simulink model "Battery"  (R2018b)
settings: Solver=VariableStepAuto  StartTime=0.0  StopTime=10.0  RelTol=1e-3
settings Model: Creator=jackb  LastModifiedBy=jackb
settings DebuggingCC: LibraryContextMissingDiagnostic=none
settings SFSimCC: SimUseLocalCustomCode=off
settings RTWCC: RTWUseLocalCustomCode=off

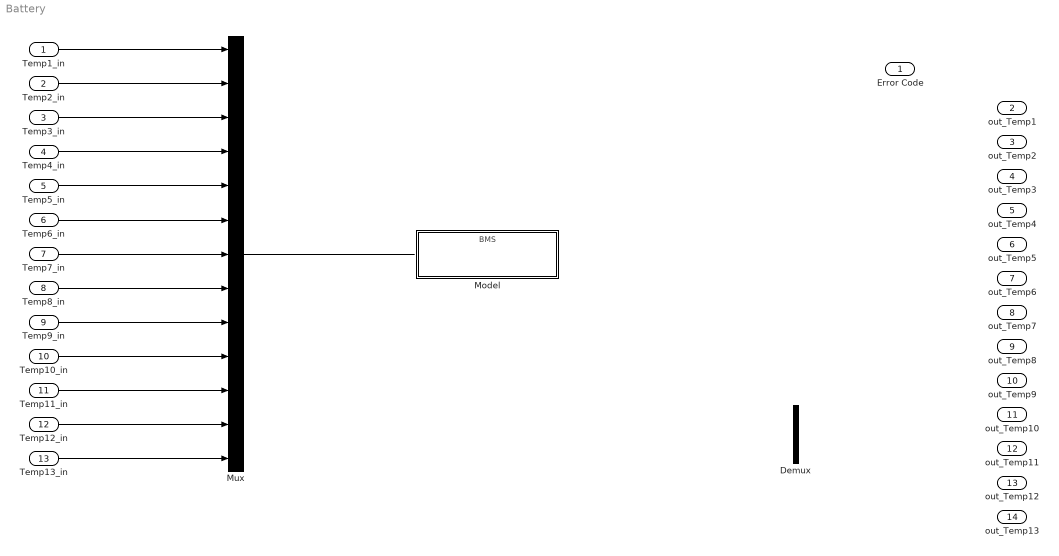
== system Battery ==
  Temp1_in : Inport
  Temp2_in : Inport  Port=2
  "Temp3_in " : Inport  Port=3
  Temp4_in : Inport  Port=4
  Temp5_in : Inport  Port=5
  Temp6_in : Inport  Port=6
  Temp7_in : Inport  Port=7
  Temp8_in : Inport  Port=8
  Temp9_in : Inport  Port=9
  Temp10_in : Inport  Port=10
  Temp11_in : Inport  Port=11
  Temp12_in : Inport  Port=12
  Temp13_in : Inport  Port=13
  Demux : Demux  Outputs=13
  Model : ModelReference  ModelNameDialog=BMS  SimulationMode=Normal
  Mux : Mux  Inputs=13
  Error Code : Outport
  out_Temp1 : Outport  Port=2
  out_Temp2 : Outport  Port=3
  out_Temp3 : Outport  Port=4
  out_Temp4 : Outport  Port=5
  out_Temp5 : Outport  Port=6
  out_Temp6 : Outport  Port=7
  out_Temp7 : Outport  Port=8
  out_Temp8 : Outport  Port=9
  out_Temp9 : Outport  Port=10
  out_Temp10 : Outport  Port=11
  out_Temp11 : Outport  Port=12
  out_Temp12 : Outport  Port=13
  out_Temp13 : Outport  Port=14
  wires:
  Temp1_in/1 -> Mux/1
  Temp2_in/1 -> Mux/2
  "Temp3_in "/1 -> Mux/3
  Temp4_in/1 -> Mux/4
  Temp5_in/1 -> Mux/5
  Temp6_in/1 -> Mux/6
  Temp7_in/1 -> Mux/7
  Temp8_in/1 -> Mux/8
  Temp9_in/1 -> Mux/9
  Temp10_in/1 -> Mux/10
  Temp11_in/1 -> Mux/11
  Temp12_in/1 -> Mux/12
  Temp13_in/1 -> Mux/13
  Mux/1 -> ?
